simulink model "BD_PAR_SS"  (Simulink 10.3)
settings: Solver=ode1  StartTime=0.0  StopTime=max(cyc_mph(:,1))  FixedStep=1  MaxStep=1  RelTol=1e-3  AbsTol=1e-3
undefined symbols (not defined in the file): acc_elec_eff, acc_elec_pwr, acc_mech_eff, amb_tmp, cs_charge_deplete_bool, cs_electric_decel_spd, cs_electric_launch_spd_hi, cs_electric_launch_spd_lo, cs_hi_soc, cs_lo_soc, cs_off_trq_frac, cyc_avg_time, cyc_cargo_mass, cyc_elevation_init, cyc_filter_bool, cyc_grade, cyc_mph, ess_module_num, ess_on, ess_voc, ex_calc, ex_cat_co_frac, ex_cat_ext_cp, ex_cat_ext_emisv, ex_cat_ext_init_tmp, ex_cat_ext_mass, ex_cat_ext_sarea, ex_cat_hc_frac, ex_cat_i2p_th_cond, ex_cat_i2x_emisv, ex_cat_i2x_th_cond, ex_cat_int_cp, ex_cat_int_init_tmp, ex_cat_int_mass, ex_cat_int_sarea, ex_cat_lim, ex_cat_m2i_th_cond, ex_cat_m2i_tmp, ex_cat_m2p_emisv, ex_cat_mon_cp, ex_cat_mon_init_tmp, ex_cat_mon_mass, ex_cat_mon_sarea, ex_cat_monf_sarea, ex_cat_moni_sarea, ex_cat_nox_frac, ex_cat_p2x_th_cond, ex_cat_pcm_ecp, ex_cat_pcm_mass, ex_cat_pcm_tmp, ex_cat_pipe_cp, ex_cat_pipe_emisv, ex_cat_pipe_init_tmp, ex_cat_pipe_mass, ex_cat_pipe_sarea, ex_cat_pm_frac, ex_cat_tmp_range, ex_gas_cp, ex_manif_cp, ex_manif_emisv ... (+73)
libraries: lib_controls x6, lib_vehicle x3, lib_accessory x2, lib_interactive x1, lib_energy_storage x1, lib_fuel_converter x1
(part 4 of 6)

== system BD_PAR_SS/motor/ controller <mc> par/motor speed estimator ==
  mc_spd_out_a : Inport
  <= max spd : Saturate  UpperLimit=max(mc_map_spd)*mc_spd_scale  LowerLimit=-inf
  Block NOTES : Subsystem
      mask Display: disp('Block\nNOTES')
  Constant : Constant  Value=eps
  Constant1 : Constant  Value=0
  Constant2 : Constant  Value=2
  Gain : Gain  Gain=0.447  SaturateOnIntegerOverflow=on
  Logical Operator1 : Logic
  Memory : Memory  InitialCondition=cyc_mph(1,2)*0.447/wh_radius*fd_ratio*max(gb_ratio)*tc_mc_to_fc_ratio
  Memory1 : Memory  InitialCondition=1
  Memory2 : Memory
  Product : Product  Inputs=**/  SaturateOnIntegerOverflow=on
  Relational : RelationalOperator  Operator=>  RndMeth=Nearest  InputSameDT=on
  Relational Operator1 : RelationalOperator  Operator=~=  RndMeth=Nearest  InputSameDT=on
  Sum : Sum  SaturateOnIntegerOverflow=on
  Sum1 : Sum  Inputs=-+  SaturateOnIntegerOverflow=on
  Switch : Switch  Threshold=eps  SaturateOnIntegerOverflow=on  InputSameDT=on
  Switch1 : Switch  Threshold=eps  SaturateOnIntegerOverflow=on  InputSameDT=on
  To Workspace7 : ToWorkspace  VariableName=mc_spd_est  SampleTime=-1
  Out1 : Outport
  tag scope: mc_spd_limited=global
  wires:
  Switch/1 -> Memory/1
  Memory1/1 -> Switch1/2
  Relational/1 -> Memory1/1
  Sum1/1 -> Relational/1
  Constant2/1 -> Relational/2
  [mpha] -> Sum1/1, Gain/1
  [cyc_mph_r] -> Sum1/2
  Constant/1 -> Sum/2
  Memory/1 -> Switch1/1
  Constant1/1 -> Switch/3
  [veh_spd_a_rec] -> Switch/2, Sum/1
  Gain/1 -> Product/2
  Sum/1 -> Product/3
  Product/1 -> Switch/1
  mc_spd_out_a/1 -> Product/1, Switch1/3
  Memory2/1 -> Logical Operator1/2
  Logical Operator1/1 -> [mc_spd_limited]
  Relational Operator1/1 -> Logical Operator1/1, Memory2/1
  Switch1/1 -> <= max spd/1, Relational Operator1/1
  <= max spd/1 -> Out1/1, To Workspace7/1, Relational Operator1/2

== system BD_PAR_SS/motor/ controller <mc> par/rotor drive torque available (Nm) ==
  torque per unit input power (N-m/W) : Inport
  available input power (W) : Inport  Port=2
  Block NOTES : Subsystem
      mask Display: disp('Block\nNOTES')
  Constant2 : Constant  Value=inf
  Constant3 : Constant  Value=0
  Product : Product  SaturateOnIntegerOverflow=on
  Relational Operator : RelationalOperator  Operator=~=  RndMeth=Nearest  InputSameDT=on
  Switch : Switch  Threshold=eps  SaturateOnIntegerOverflow=on  InputSameDT=on
  rotor drive torque available : Outport  InitialOutput=0
  wires:
  torque per unit input power (N-m/W)/1 -> Relational Operator/1, Product/1
  Switch/1 -> rotor drive torque available/1
  Relational Operator/1 -> Switch/2
  Product/1 -> Switch/1
  available input power (W)/1 -> Product/2
  Constant2/1 -> Relational Operator/2
  Constant3/1 -> Switch/3

== system BD_PAR_SS/power bus <pb>/Block NOTES ==
  note: This power bus requires power from (or distributes power to)
      | the generator first, taking the balance from the energy
      | storage system.

== system BD_PAR_SS/torque coupler <tc>/Block NOTES ==
  note: speed, while the motor's speed may be different.  The ratio of motor speed to main
      | output speed is stored in the variable tc_mc_to_fc_spd_ratio.
  note: This block models a chain- or belt-driven torque coupler, with three gears:  one each
      | for the motor, main input (the engine or gearbox), and main output (to the gearbox
      | or final drive).  It includes losses in the chain or belt, but leaves inertia effects to be
      | considered in the appropriate component.
      |
      | The entire torque required out of the torque coupler (plus losses) is required from the
      | engine.  The engine provides only as much torque as its engine controller (see the
      | <vc> block) allows.  Any remaining unmet torque request is submitted to the motor,
      | which meets the request to the best of its ability.
      |
      | The torque converter output speed is limited by the maximum speeds of both the
      | motor and the engine.
      |
      | The loss torque is zero when the gears are not turning, and is applied at the output
      |  gear.
      |
      | The gears connecting the main input and main output to the torque converter's belt
      | or chain are assumed to be of the same size, so that main input speed = main output

== system BD_PAR_SS/torque coupler <tc>/help ==

== system BD_PAR_SS/torque coupler <tc>/loss (Nm) ==
  note: The loss torque is zero when the gears are not turning,
      | and is applied at the torque coupler's output gear.
  tc output speed (rad/s) : Inport
  Constant : Constant  Value=0
  Switch : Switch  Threshold=eps  SaturateOnIntegerOverflow=on  InputSameDT=on
  torque coupler loss torque (Nm) : Constant  Value=tc_loss
  drag torque (Nm) : Outport  InitialOutput=0
  wires:
  torque coupler loss torque (Nm)/1 -> Switch/1
  Switch/1 -> drag torque (Nm)/1
  tc output speed (rad/s)/1 -> Switch/2
  Constant/1 -> Switch/3

== system BD_PAR_SS/vehicle <veh>/Block NOTES ==
  note: A slight simplification, the assumption that (speed_at_end_of_time_step)^2 is roughly equal to
      | (speed_at_end_of_time_step)*(speed_at_beginning_of_time_step), is used to avoid solving
      | a quadratic equation in the solution of v=v(Ftract).
  note: This block uses the required vehicle speed with vehicle parameters and the previous speed
      | and classic, straightforward equations to determine the tractive force required at the tire/road interface.
  note: If no drivetrain component ran up against its performance limit during the time step, the achieved speed
      | is taken to be the requested speed.
  note: Given the tractive force available, this block uses the same equations to determine the achievable speed.

== system BD_PAR_SS/vehicle <veh>/force req'd to accelerate (N) ==
  v(m/s) : Inport
  v prev : Inport  Port=2
  Clock : Clock
  Memory : Memory  InitialCondition=-0.1
  Product1 : Product  Inputs=**/  SaturateOnIntegerOverflow=on
  Sum : Sum  Inputs=+-  SaturateOnIntegerOverflow=on
  Sum1 : Sum  Inputs=+-  SaturateOnIntegerOverflow=on
  current veh mass : Subsystem
  (N) : Outport  InitialOutput=0
  wires:
  current veh mass/1(Out1) -> Product1/1
  Clock/1 -> Sum1/1, Memory/1
  Memory/1 -> Sum1/2
  Product1/1 -> (N)/1
  v prev/1 -> Sum/2
  v(m/s)/1 -> Sum/1
  Sum1/1 -> Product1/3
  Sum/1 -> Product1/2

== system BD_PAR_SS/vehicle <veh>/force req'd to ascend (N) ==
  average vehicle speed over time step (m/s) : Inport
  Constant : Constant  Value=veh_gravity
  Constant1 : Constant  Value=0
  Product : Product  Inputs=3  SaturateOnIntegerOverflow=on
  Switch : Switch  SaturateOnIntegerOverflow=on  InputSameDT=on
  Trigonometric Function : Trigonometry  Operator=atan
  Trigonometric Function1 : Trigonometry
  current veh mass : Subsystem
  (N) : Outport  InitialOutput=0
  wires:
  current veh mass/1(Out1) -> Product/3
  average vehicle speed over time step (m/s)/1 -> Switch/2
  Constant1/1 -> Switch/3
  Switch/1 -> (N)/1
  Product/1 -> Switch/1
  Constant/1 -> Product/1
  [grade] -> Trigonometric Function/1
  Trigonometric Function1/1 -> Product/2
  Trigonometric Function/1 -> Trigonometric Function1/1

== system BD_PAR_SS/vehicle <veh>/force req'd to overcome aerodynamic drag (N) ==
  average vehicle speed over time step (m/s) : Inport
  Constant : Constant  Value=veh_air_density*veh_CD*veh_FA*0.5
  Product : Product  Inputs=3  SaturateOnIntegerOverflow=on
  D aero(N) : Outport  InitialOutput=0
  wires:
  Product/1 -> D aero(N)/1
  Constant/1 -> Product/3
  average vehicle speed over time step (m/s)/1 -> Product/2, Product/1

== system BD_PAR_SS/vehicle <veh>/help ==

== system BD_PAR_SS/vehicle <veh>/record achieved force outputs ==
  spd_prev : Inport
  spd : Inport  Port=2
  Gain1 : Gain  Gain=0.5  SaturateOnIntegerOverflow=on
  Product{,1..3} (4 alike) : Product  SaturateOnIntegerOverflow=on
  Sum2 : Sum  SaturateOnIntegerOverflow=on
  To Workspace1 : ToWorkspace  VariableName=veh_pwr_rr_a  SampleTime=-1
  To Workspace4 : ToWorkspace  VariableName=veh_pwr_accel_a  SampleTime=-1
  To Workspace6 : ToWorkspace  VariableName=veh_pwr_drag_a  SampleTime=-1
  To Workspace7 : ToWorkspace  VariableName=veh_pwr_ascent_a  SampleTime=-1
  force req'd to accelerate (N)1 : Subsystem
  force req'd to ascend (N)1 : Subsystem
  force req'd to overcome aerodynamic drag (N)1 : Subsystem
  rolling resistance force : Subsystem  BlockChoice=force req'd to overcome rolling resistance (N)
      settings: AttributesFormatString=%<BlockChoice>  TemplateBlock=lib_vehicle/Submodels/rolling resistance force  MemberBlocks=force req'd to overcome rolling resistance (N),force req'd to overcome rolling resistance (N) j2452
  tag scope: veh_pwr_accel_a=global, veh_pwr_ascent_a=global, veh_pwr_drag_a=global, veh_pwr_rr_a=global
  wires:
  Gain1/1 -> [vel_ave], rolling resistance force/1(average vehicle speed over time step (m/s)), force req'd to ascend (N)1/1(average vehicle speed over time step (m/s)), force req'd to overcome aerodynamic drag (N)1/1(average vehicle speed over time step (m/s))
  Product3/1 -> To Workspace1/1, [veh_pwr_rr_a]
  [vel_ave] -> Product3/2
  Product2/1 -> [veh_pwr_ascent_a], To Workspace7/1
  [vel_ave] -> Product2/2
  [vel_ave] -> Product1/2
  [vel_ave] -> Product/2
  Product1/1 -> [veh_pwr_drag_a], To Workspace6/1
  Product/1 -> [veh_pwr_accel_a], To Workspace4/1
  force req'd to accelerate (N)1/1((N)) -> Product/1
  rolling resistance force/1(Fr (N)) -> Product3/1
  force req'd to ascend (N)1/1((N)) -> Product2/1
  force req'd to overcome aerodynamic drag (N)1/1(D aero(N)) -> Product1/1
  spd_prev/1 -> Sum2/2, force req'd to accelerate (N)1/2(v prev)
  spd/1 -> Sum2/1, force req'd to accelerate (N)1/1(v(m/s))
  Sum2/1 -> Gain1/1

== system BD_PAR_SS/vehicle <veh>/rolling resistance force ==
  average vehicle speed over time step (m/s) : Inport
  force req'd to overcome rolling resistance (N) : lib_vehicle/Submodels/force req'd to overcome rolling resistance (N)  SystemSampleTime=-1  VariantActivationTime=update diagram  Latency=0  AutoFrameSizeCalculation=off
  Fr (N) : Outport
  wires:
  average vehicle speed over time step (m/s)/1 -> force req'd to overcome rolling resistance (N)/1
  force req'd to overcome rolling resistance (N)/1 -> Fr (N)/1

== system BD_PAR_SS/vehicle <veh>/vehicle speed ==
  vehicle speed at beginning of time step (m/s) : Inport
  "available tractive force and linear speed (N), (m/s)" : Inport  Port=2
  vehicle speed (m/s) : lib_vehicle/Submodels/vehicle speed (m//s)  SystemSampleTime=-1  VariantActivationTime=update diagram  Latency=0  AutoFrameSizeCalculation=off
  vehicle speed achievable at end of time step (m/s) : Outport
  wires:
  vehicle speed at beginning of time step (m/s)/1 -> vehicle speed (m/s)/1
  "available tractive force and linear speed (N), (m/s)"/1 -> vehicle speed (m/s)/2
  vehicle speed (m/s)/1 -> vehicle speed achievable at end of time step (m/s)/1

== system BD_PAR_SS/wheel and axle  front/rear <wh>/Block NOTES ==
  note: This block determines the required axle torque and speed given the tractive force and
      | speed required to meet the trace in the top blocks, and determines the available tractive
      | force and possible vehicle speed given the drivetrain-input torque and rotational speed
      | in the bottom blocks.  The "wheel control" blocks apply the braking strategy and ensure
      | that accelerations beyond the capability of the tires are not requested.

== system BD_PAR_SS/wheel and axle  front/rear <wh>/effect of  inertia (Nm) ==
  note: This block computes the torque required to overcome the inertia of the
      | wheels and axle.
  axle input speed (rad/s) : Inport
  Constant : Constant  Value=wh_inertia
  Product : Product  SaturateOnIntegerOverflow=on
  d/dt : Derivative
  inertia torque (Nm) : Outport  InitialOutput=0
  wires:
  Product/1 -> inertia torque (Nm)/1
  Constant/1 -> Product/2
  axle input speed (rad/s)/1 -> d/dt/1
  d/dt/1 -> Product/1

== system BD_PAR_SS/wheel and axle  front/rear <wh>/front brake ==
  F_brake : Inport
  Constant : Constant  Value=wh_max_front_brake_force
  Terminator : Terminator
  F_brake_max : Outport  InitialOutput=0
  wires:
  Constant/1 -> F_brake_max/1
  F_brake/1 -> Terminator/1

== system BD_PAR_SS/wheel and axle  front/rear <wh>/front force ==
  In1 : Inport
  In2 : Inport  Port=2
  Product1 : Product  SaturateOnIntegerOverflow=on
  Sum2 : Sum  Inputs=-+  SaturateOnIntegerOverflow=on
  To Workspace12 : ToWorkspace  VariableName=wh_front_brake_r  SampleTime=-1
  brake request  controller interface : Subsystem
  tractive torque req/d of drivetrain (Nm) : Gain  Gain=wh_radius  SaturateOnIntegerOverflow=on
  Out1 : Outport
  wires:
  tractive torque req/d of drivetrain (Nm)/1 -> Out1/1
  In2/1 -> Product1/2
  In1/1 -> Product1/1
  Product1/1 -> Sum2/2
  Sum2/1 -> tractive torque req/d of drivetrain (Nm)/1
  brake request  controller interface/1(F_front_brake_req) -> To Workspace12/1, Sum2/1

== system BD_PAR_SS/wheel and axle  front/rear <wh>/front/rear brake controller interface (achievable) ==
  F_drivetrain_ach : Inport
  w_wheel_ach : Inport  Port=2
  F_rear_drivetrain_ach : Inport  Port=3
  F_max_front_brake : Inport  Port=4
  F_max_rear_brake : Inport  Port=5
  F_front_brake : Outport  InitialOutput=0
  F_rear_brake : Outport  Port=2  InitialOutput=0
  tag scope: F_drivetrain_ach=global, F_max_front_brake=global, F_max_rear_brake=global, F_rear_drivetrain_ach=global, w_wheel_ach=global
  wires:
  F_rear_drivetrain_ach/1 -> [F_rear_drivetrain_ach]
  F_max_rear_brake/1 -> [F_max_rear_brake]
  F_max_front_brake/1 -> [F_max_front_brake]
  F_drivetrain_ach/1 -> [F_drivetrain_ach]
  w_wheel_ach/1 -> [w_wheel_ach]
  [F_front_brake] -> F_front_brake/1
  [F_rear_brake] -> F_rear_brake/1

== system BD_PAR_SS/wheel and axle  front/rear <wh>/help ==

== system BD_PAR_SS/wheel and axle  front/rear <wh>/limits and losses diagnostics ==
  speed : Inport
  front brake : Inport  Port=2
  front brake max : Inport  Port=3
  rear brake max : Inport  Port=4
  rear brake : Inport  Port=5
  Gain : Gain  Gain=-1  SaturateOnIntegerOverflow=on
  Logical Operator : Logic  Operator=OR
  Product : Product  SaturateOnIntegerOverflow=on
  Relational Operator1 : RelationalOperator  Operator===  RndMeth=Nearest  InputSameDT=on
  Relational Operator2 : RelationalOperator  Operator===  RndMeth=Nearest  InputSameDT=on
  Sum3 : Sum  SaturateOnIntegerOverflow=on
  To Workspace6 : ToWorkspace  VariableName=wh_brake_loss_pwr  SampleTime=-1
  tag scope: brake_limited=global
  wires:
  rear brake/1 -> Relational Operator2/2, Sum3/2
  rear brake max/1 -> Relational Operator2/1
  front brake max/1 -> Relational Operator1/2
  front brake/1 -> Relational Operator1/1, Sum3/1
  speed/1 -> Product/1
  Relational Operator2/1 -> Logical Operator/2
  Relational Operator1/1 -> Logical Operator/1
  Logical Operator/1 -> [brake_limited]
  Product/1 -> To Workspace6/1
  Sum3/1 -> Gain/1
  Gain/1 -> Product/2

== system BD_PAR_SS/wheel and axle  front/rear <wh>/loss (Nm) ==
  note: The loss torque is zero when the axle is not turning.
  axle speed (rad/s) : Inport
  Constant : Constant  Value=0
  Switch : Switch  Threshold=eps  SaturateOnIntegerOverflow=on  InputSameDT=on
  veh mass calc : Subsystem
  wheel & axle bearing drag (Nm) : Lookup  InputValues=wh_axle_loss_mass  Table=wh_axle_loss_trq  SaturateOnIntegerOverflow=on
  drag torque (Nm) : Outport  InitialOutput=0
  wires:
  wheel & axle bearing drag (Nm)/1 -> Switch/1
  Constant/1 -> Switch/3
  axle speed (rad/s)/1 -> Switch/2
  Switch/1 -> drag torque (Nm)/1
  veh mass calc/1(Out1) -> wheel & axle bearing drag (Nm)/1

== system BD_PAR_SS/wheel and axle  front/rear <wh>/rear brake ==
  F_brake : Inport
  Constant : Constant  Value=wh_max_rear_brake_force
  Terminator : Terminator
  F_brake_max : Outport  InitialOutput=0
  wires:
  F_brake/1 -> Terminator/1
  Constant/1 -> F_brake_max/1

== system BD_PAR_SS/wheel and axle  front/rear <wh>/rear force ==
  In1 : Inport
  In2 : Inport  Port=2
  Product2 : Product  SaturateOnIntegerOverflow=on
  Sum1 : Sum  Inputs=-+  SaturateOnIntegerOverflow=on
  Sum4 : Sum  Inputs=-+  SaturateOnIntegerOverflow=on
  To Workspace12 : ToWorkspace  VariableName=wh_rear_brake_r  SampleTime=-1
  brake request controller interface1 : Subsystem
  tractive torque req/d of drivetrain (Nm)1 : Gain  Gain=wh_radius  SaturateOnIntegerOverflow=on
  Out1 : Outport
  wires:
  Sum1/1 -> Sum4/2
  Product2/1 -> Sum1/1
  In2/1 -> Product2/2
  In1/1 -> Sum1/2, Product2/1
  tractive torque req/d of drivetrain (Nm)1/1 -> Out1/1
  Sum4/1 -> tractive torque req/d of drivetrain (Nm)1/1
  brake request controller interface1/1(F_rear_brake_req) -> To Workspace12/1, Sum4/1

== system BD_PAR_SS/wheel and axle  front/rear <wh>/tire slip model (m/s) ==
  note: See note regarding sum in backward path
  weight borne  by front axle (N) : Inport
  total tractive  force available (N) : Inport  Port=2
  axle speed available (rad/s) : Inport  Port=3
  axle speed req'd (rad/s) : Inport  Port=4
  vehicle speed required (m/s) : Inport  Port=5
  weight borne by  rear axle (N) : Inport  Port=6
  front fraction : Inport  Port=7
  Abs1 : Abs  SaturateOnIntegerOverflow=on
  Block NOTES : Subsystem
      mask Display: disp('Block\nNOTES')
  Constant : Constant  Value=1e-3
  Constant5 : Constant
  Constant6 : Constant  Value=wh_radius
  Fcn : Fcn  Expr=1/u
  Relational Operator1 : RelationalOperator  Operator=>  RndMeth=Nearest  InputSameDT=on
  Sum1 : Sum  Inputs=+-  SaturateOnIntegerOverflow=on
  Sum2 : Sum  SaturateOnIntegerOverflow=on
  Sum3 : Sum  SaturateOnIntegerOverflow=on
  Sum4 : Sum  Inputs=-+  SaturateOnIntegerOverflow=on
  Switch1 : Switch  Threshold=eps  SaturateOnIntegerOverflow=on  InputSameDT=on
  front axle : Subsystem
  front frac : Product  SaturateOnIntegerOverflow=on
  rear axle : Subsystem
  vehicle speed (m/s) : Product  Inputs=3  SaturateOnIntegerOverflow=on
  possible vehicle speed (m/s) : Outport  InitialOutput=0
  tag scope: veh_spd_a_rec=global
  wires:
  Sum2/1 -> Sum3/1
  rear axle/1(Out1) -> Sum2/2
  front axle/1(Out1) -> Sum2/1
  Sum1/1 -> rear axle/2(In2)
  front frac/1 -> Sum1/2, front axle/2(In2)
  front fraction/1 -> front frac/2
  total tractive  force available (N)/1 -> Sum1/1, front frac/1
  weight borne by  rear axle (N)/1 -> rear axle/1(In1)
  vehicle speed (m/s)/1 -> [veh_spd_a_rec], Switch1/1
  Switch1/1 -> possible vehicle speed (m/s)/1
  weight borne  by front axle (N)/1 -> front axle/1(In1)
  Abs1/1 -> Relational Operator1/1
  Constant/1 -> Relational Operator1/2
  axle speed req'd (rad/s)/1 -> Sum4/2
  Sum4/1 -> Abs1/1
  vehicle speed required (m/s)/1 -> Switch1/3
  Relational Operator1/1 -> Switch1/2
  Constant6/1 -> vehicle speed (m/s)/3
  axle speed available (rad/s)/1 -> vehicle speed (m/s)/2, Sum4/1
  Constant5/1 -> Sum3/2
  Fcn/1 -> vehicle speed (m/s)/1
  Sum3/1 -> Fcn/1

== system BD_PAR_SS/wheel and axle  front/rear <wh>/tire slip model (rad/s) ==
  note: Question: for front and rear, is it the sum of or min/max? tm:020703
  note: This block implements the effects of finite tire slip
      | (with respect to the road) on the vehicle speed/wheel speed relationship.
  note: Slip is defined as s=(omega*r - v) / v.  The one-to-one mapping of slip to normalized
      | tractive force, F_tract/W_front_axle, up to the maximum, is stored in the variables
      | "wh_slip" and "wh_slip_force_coeff."
  total tractive  force requested (N) : Inport
  requested time-step average vehicle speed (m/s) : Inport  Port=2
  weight borne by front axle (N) : Inport  Port=3
  weight borne by  rear axle (N)1 : Inport  Port=4
  front traction ratio : Inport  Port=5
  Constant5 : Constant
  Constant6 : Constant  Value=1/wh_radius
  Sum1 : Sum  Inputs=+-  SaturateOnIntegerOverflow=on
  Sum2 : Sum  SaturateOnIntegerOverflow=on
  Sum3 : Sum  SaturateOnIntegerOverflow=on
  To Workspace6 : ToWorkspace  VariableName=wh_slip_r  SampleTime=-1
  front frac : Product  SaturateOnIntegerOverflow=on
  front slip : Subsystem
  rear slip : Subsystem
  wheel speed (rad/s) : Product  Inputs=3  SaturateOnIntegerOverflow=on
  slip-augmented rotational speed (rad/s) : Outport  InitialOutput=0
  wires:
  Sum2/1 -> To Workspace6/1, Sum3/1
  rear slip/1(Out1) -> Sum2/2
  front slip/1(Out1) -> Sum2/1
  weight borne by  rear axle (N)1/1 -> rear slip/1(In1)
  Sum1/1 -> rear slip/2(In2)
  front traction ratio/1 -> front frac/2
  total tractive  force requested (N)/1 -> Sum1/1, front frac/1
  front frac/1 -> front slip/2(In2), Sum1/2
  wheel speed (rad/s)/1 -> slip-augmented rotational speed (rad/s)/1
  Constant5/1 -> Sum3/2
  Sum3/1 -> wheel speed (rad/s)/2
  Constant6/1 -> wheel speed (rad/s)/3
  requested time-step average vehicle speed (m/s)/1 -> wheel speed (rad/s)/1
  weight borne by front axle (N)/1 -> front slip/1(In1)

== system BD_PAR_SS/wheel and axle  front/rear <wh>/traction controller interface ==
  F_req : Inport
  v_ave_req : Inport  Port=2
  F_req_limited : Outport  InitialOutput=0
  v_req_limited : Outport  Port=2  InitialOutput=0
  wt_front_axle : Outport  Port=3  InitialOutput=0
  wt_rear_axle : Outport  Port=4  InitialOutput=0
  front_traction_ratio : Outport  Port=5  InitialOutput=0
  tag scope: F_req=global, v_ave_req=global
  wires:
  [front_traction_ratio] -> front_traction_ratio/1
  [wt_rear_axle] -> wt_rear_axle/1
  v_ave_req/1 -> [v_ave_req]
  F_req/1 -> [F_req]
  [wt_front_axle] -> wt_front_axle/1
  [v_req_limited] -> v_req_limited/1
  [F_req_limited] -> F_req_limited/1

== system BD_PAR_SS/<vc> par/engine on (parallel hybrid)/Block NOTES1 ==
  note: This engine state computer keeps the engine on if:
      | [
      | 1) key is on, AND
      | 2) (trq is too high AND speed is too high for idle) OR engine is allowed to idle, AND
      | 3) vehicle speed >= cs_electric_launch_spd [ in m/s ], AND
      | 4) req'd trq > (cs_off_trq_frac * max_trq_at_spd) OR SOC<cs_lo_soc
      | ]
      | OR
      | [ engine was previously on AND the transmission is shifting ]
      |
      | The last condition is added to prevent the engine from unrealistically
      | shutting down for a second or two during a shift.

== system BD_PAR_SS/<vc> par/engine on (parallel hybrid)/Subsystem ==
  in_1 : Inport
  Clock : Clock
  Constant1 : Constant  Value=n
  Constant2 : Constant
  Integrator : Integrator
  Memory : Memory  InitialCondition=-0.1
  Memory1 : Memory
  Product : Product  Inputs=*/  InputSameDT=on  RndMeth=Zero  SaturateOnIntegerOverflow=on  OutDataTypeStr=Inherit: Same as first input
  Product1 : Product  InputSameDT=on  RndMeth=Zero  SaturateOnIntegerOverflow=on  OutDataTypeStr=Inherit: Same as first input
  Relational Operator : RelationalOperator  Operator=<=  RndMeth=Nearest  InputSameDT=on
  Sum : Sum  Inputs=+-  InputSameDT=on  SaturateOnIntegerOverflow=on  OutDataTypeStr=Inherit: Same as first input
  Sum1 : Sum  Inputs=|+-  InputSameDT=on  SaturateOnIntegerOverflow=on  OutDataTypeStr=Inherit: Same as first input
  Switch{,1..3} (4 alike) : Switch  Threshold=eps  SaturateOnIntegerOverflow=on  InputSameDT=on
  Variable Transport Delay : VariableTransportDelay  MaximumDelay=n  ZeroDelay=on
  out_1 : Outport  InitialOutput=0
  wires:
  Product/1 -> out_1/1
  Sum/1 -> Product/1
  Variable Transport Delay/1 -> Sum/2
  Integrator/1 -> Variable Transport Delay/1, Sum/1
  Relational Operator/1 -> Switch/2
  Constant1/1 -> Product1/2
  Clock/1 -> Sum1/1, Memory/1, Relational Operator/1, Switch/1
  Memory/1 -> Sum1/2
  Sum1/1 -> Product1/1
  Product1/1 -> Relational Operator/2, Switch/3
  Switch/1 -> Variable Transport Delay/2, Switch1/2, Switch1/1
  Constant2/1 -> Switch1/3
  Switch1/1 -> Product/2
  Switch2/1 -> Integrator/1
  Switch3/1 -> Memory1/1
  in_1/1 -> Switch2/3, Switch3/3
  Memory1/1 -> Switch2/1, Switch3/1
  [shifting] -> Switch2/2, Switch3/2

== system BD_PAR_SS/<vc> par/engine on (parallel hybrid)/key_on ==
  Clock : Clock
  Fcn1 : Fcn  Expr=rem(u[1],period)
  Look-Up Table : Lookup  InputValues=t  Table=y  SaturateOnIntegerOverflow=on
  out_1 : Outport  InitialOutput=0
  wires:
  Fcn1/1 -> Look-Up Table/1
  Clock/1 -> Fcn1/1
  Look-Up Table/1 -> out_1/1

== system BD_PAR_SS/<vc> par/engine on (parallel hybrid)/repeated cycle:  speed required at end of NEXT step ==
  Clock : Clock
  Fcn1 : Fcn  Expr=rem(u[1],period)
  Look-Up Table : Lookup  InputValues=t  Table=y  SaturateOnIntegerOverflow=on
  Memory : Memory  InitialCondition=-0.1
  Sum : Sum  Inputs=+-  InputSameDT=on  SaturateOnIntegerOverflow=on  OutDataTypeStr=Inherit: Same as first input
  Sum1 : Sum  InputSameDT=on  SaturateOnIntegerOverflow=on  OutDataTypeStr=Inherit: Same as first input
  out_1 : Outport  InitialOutput=0
  wires:
  Sum1/1 -> Look-Up Table/1
  Look-Up Table/1 -> out_1/1
  Fcn1/1 -> Sum1/1
  Sum/1 -> Sum1/2
  Memory/1 -> Sum/2
  Clock/1 -> Fcn1/1, Memory/1, Sum/1

== system BD_PAR_SS/<vc> par/motor controller logic/Block NOTES ==
  note: This block models a motor/controller's logic, modulating the power input requirement as follows:
      | - enforcing the maximum current limit of the motor/controller
      | - shutting the motor off if the average speed over the time step ==0
      | - shutting the motor off if the transmission is shifting.

== system BD_PAR_SS/<vc> par/motor controller logic/Sign ==
  in_1 : Inport
  Constant : Constant  Value=0
  Relational Operator : RelationalOperator  Operator=>  RndMeth=Nearest  InputSameDT=on
  Relational Operator1 : RelationalOperator  Operator=<  RndMeth=Nearest  InputSameDT=on
  Sum : Sum  Inputs=+-  InputSameDT=on  SaturateOnIntegerOverflow=on  OutDataTypeStr=Inherit: Same as first input
  out_1 : Outport  InitialOutput=0
  wires:
  Sum/1 -> out_1/1
  Relational Operator/1 -> Sum/1
  Relational Operator1/1 -> Sum/2
  Constant/1 -> Relational Operator/2, Relational Operator1/2
  in_1/1 -> Relational Operator1/1, Relational Operator/1

== system BD_PAR_SS/<vc> par/parallel clutch control/Block NOTES ==
  note: This clutch control block determines the clutch state given the req'd clutch output torque
      | and speed (labelled as gearbox input torque and speed), and the gear number history.
      |                           conditions                                                                       clutch state
      | gear is being shifted OR (trq <~ 0 AND (engine is                                     1 == disengaged
      | clutched to avoid compression braking OR spd < idle))
      |
      | (trq >~ 0) AND (spd < launch speed) AND clutch                                       2 == slipping
      | was not engaged during previous time step
      |
      | neither of above sets of conditions are met                                          3 == engaged
      |
      | But the clutch is always disengaged when the engine is off or was off within the past 0.5 s.

== system BD_PAR_SS/<vc> par/parallel clutch control/gearbox speed estimator ==
  gb_spd_in_r if no gear change : Inport
  Block NOTES : Subsystem
      mask Display: disp('Block\nNOTES')
  Constant : Constant  Value=eps
  Constant1 : Constant  Value=0
  Constant2 : Constant
  Constant3 : Constant  Value=0.11
  Gain : Gain  Gain=0.447  SaturateOnIntegerOverflow=on  OutDataTypeStr=Inherit: Same as input  ParamDataTypeStr=Inherit: Same as input
  Logical : Logic
  Memory : Memory  InitialCondition=cyc_mph(1,2)*0.447/wh_radius*fd_ratio*gb_ratio(gb_num_init)
  Memory1 : Memory  InitialCondition=1
  Product : Product  Inputs=**/  InputSameDT=on  RndMeth=Zero  SaturateOnIntegerOverflow=on  OutDataTypeStr=Inherit: Same as first input
  Relational : RelationalOperator  Operator=>  RndMeth=Nearest  InputSameDT=on
  Relational1 : RelationalOperator  Operator=<=  RndMeth=Nearest  InputSameDT=on
  Sum : Sum  InputSameDT=on  SaturateOnIntegerOverflow=on  OutDataTypeStr=Inherit: Same as first input
  Sum1 : Sum  Inputs=-+  InputSameDT=on  SaturateOnIntegerOverflow=on  OutDataTypeStr=Inherit: Same as first input
  Switch : Switch  Threshold=eps  SaturateOnIntegerOverflow=on  InputSameDT=on
  Switch1 : Switch  Threshold=eps  SaturateOnIntegerOverflow=on  InputSameDT=on
  dt : Subsystem
  Out1 : Outport
  wires:
  Product/1 -> Switch/1
  Sum/1 -> Product/3
  Gain/1 -> Product/2
  [veh_spd_a_rec] -> Sum/1, Switch/2
  Constant1/1 -> Switch/3
  Memory/1 -> Switch1/1
  Constant/1 -> Sum/2
  [cyc_mph_r] -> Sum1/2
  [mpha] -> Gain/1, Sum1/1
  Constant2/1 -> Relational/2
  Sum1/1 -> Relational/1
  Relational/1 -> Memory1/1
  Switch/1 -> Memory/1
  Switch1/1 -> Out1/1
  gb_spd_in_r if no gear change/1 -> Switch1/3
  [gb_spd_in_a] -> Product/1
  Constant3/1 -> Relational1/2
  Relational1/1 -> Logical/2
  Memory1/1 -> Logical/1
  Logical/1 -> Switch1/2
  dt/1(Out1) -> Relational1/1

== system BD_PAR_SS/<vc> par/pre-TX parallel gearbox control/Block NOTES ==
  note: This gearbox control block computes the current gear number given the gearbox's
      | req'd output torque and speed and an estimate its efficiency.  Upshifts occur, given a
      | certain engine speed,  when the estimated engine load falls below the upshift curve
      | in engine speed/load space, and downshifts likewise occur when estimated engine
      | load rises above the downshift curve.  Separate upshift and downshift curves are
      | defined for each gear.  An upshift may not be immediately followed by a downshift.
      | If the tires are about to slip, don't upshift unless the engine would be at max. speed.
      | Enforce this rule by setting the load to 1 when the tires are about to slip.

== system BD_PAR_SS/<vc> par/pre-TX parallel gearbox control/allow downshift? ==
  prev gearnum : Inport
  Logical Operator : Logic  Operator=NOR
  Memory : Memory  InitialCondition=1
  Memory1 : Memory  InitialCondition=1
  Relational Operator1 : RelationalOperator  Operator=>  RndMeth=Nearest  InputSameDT=on
  Relational Operator2 : RelationalOperator  Operator=>  RndMeth=Nearest  InputSameDT=on
  allow shift : Outport  InitialOutput=0
  wires:
  Logical Operator/1 -> allow shift/1
  prev gearnum/1 -> Relational Operator1/1, Memory/1, Relational Operator2/1
  Relational Operator1/1 -> Logical Operator/1
  Memory/1 -> Relational Operator1/2, Memory1/1
  Memory1/1 -> Relational Operator2/2
  Relational Operator2/1 -> Logical Operator/2

== system BD_PAR_SS/<vc> par/pre-TX parallel gearbox control/allow upshift? ==
  prev gearnum : Inport
  gb_trq_out_r : Inport  Port=2
  gb_spd_out_r : Inport  Port=3
  prev Pout/Pin : Inport  Port=4
  Block NOTES1 : Subsystem
      mask Display: disp('Block\nNOTES')
  Constant : Constant
  Constant1 : Constant  Value=max(mc_map_spd)*mc_spd_scale/tc_mc_to_fc_ratio*.95
  Logical Operator1 : Logic  Operator=OR  Inputs=3
  Memory : Memory  InitialCondition=1
  Product : Product  InputSameDT=on  RndMeth=Zero  SaturateOnIntegerOverflow=on  OutDataTypeStr=Inherit: Same as first input
  Relational Operator : RelationalOperator  Operator=>  RndMeth=Nearest  InputSameDT=on
  Relational Operator1 : RelationalOperator  Operator=>  RndMeth=Nearest  InputSameDT=on
  Saturation : Saturate  UpperLimit=gb_gears_num  LowerLimit=1
  Sum : Sum  InputSameDT=on  SaturateOnIntegerOverflow=on  OutDataTypeStr=Inherit: Same as first input
  est. req'd input pwr (W) : Product  Inputs=**/  InputSameDT=on  RndMeth=Zero  SaturateOnIntegerOverflow=on  OutDataTypeStr=Inherit: Same as first input
  gear ratio : Lookup  InputValues=[1:length(gb_ratio)]  Table=gb_ratio  SaturateOnIntegerOverflow=on
  gear ratio1 : Lookup  InputValues=[1:length(gb_ratio)]  Table=gb_ratio  SaturateOnIntegerOverflow=on
  motor torque capability : Lookup  InputValues=mc_map_spd*mc_spd_scale  Table=mc_max_trq*mc_trq_scale*mc_overtrq_factor+eps  SaturateOnIntegerOverflow=on
  motor (input to gb) pwr capability : Product  InputSameDT=on  RndMeth=Zero  SaturateOnIntegerOverflow=on  OutDataTypeStr=Inherit: Same as first input
  req'd input spd if no gear change : Product  InputSameDT=on  RndMeth=Zero  SaturateOnIntegerOverflow=on  OutDataTypeStr=Inherit: Same as first input
  allow shift : Outport  InitialOutput=0
  wires:
  req'd input spd if no gear change/1 -> Relational Operator1/1
  Constant1/1 -> Relational Operator1/2
  Relational Operator1/1 -> Logical Operator1/3
  gb_spd_out_r/1 -> req'd input spd if no gear change/2, Product/2, est. req'd input pwr (W)/1
  prev gearnum/1 -> gear ratio1/1, Sum/1
  gear ratio1/1 -> req'd input spd if no gear change/1
  Constant/1 -> Sum/2
  Sum/1 -> Saturation/1
  Saturation/1 -> gear ratio/1
  gear ratio/1 -> Product/1
  motor torque capability/1 -> motor (input to gb) pwr capability/2
  Product/1 -> motor torque capability/1, motor (input to gb) pwr capability/1
  motor (input to gb) pwr capability/1 -> Relational Operator/1
  est. req'd input pwr (W)/1 -> Relational Operator/2
  gb_trq_out_r/1 -> est. req'd input pwr (W)/2
  prev Pout/Pin/1 -> est. req'd input pwr (W)/3
  Logical Operator1/1 -> allow shift/1
  Relational Operator/1 -> Logical Operator1/1
  [engine_on] -> Memory/1
  Memory/1 -> Logical Operator1/2

== system BD_PAR_SS/<vc> par/pre-TX parallel gearbox control/downshift  command ==
  prev gear number : Inport
  engine load : Inport  Port=2
  engine speed : Inport  Port=3
  Mux : Mux  Inputs=2
  Relational Operator : RelationalOperator  Operator=>  RndMeth=Nearest  InputSameDT=on
  load fraction : Subsystem  mask(Gear Selector){spd=gb_dnshift_spd, load=gb_dnshift_load}
      mask prompts: spd "Speeds:"; load "Load Fractions:"
      mask help:
      | This block will perform a linear interplation (extrapolation outside of bounds) to determine the shift point load fraction associated with the current gear number and speed.
      |
      | The Speeds parameter should be defined as an array of vectors containing speeds for each gear number.  The Load Fractions parameter should be defined as a array of vectors containing load fractions indexed by the speeds in the Speeds parameter for each gear number.
      mask Help:
      | Reference the base workspace variables - gb_**shift_spd and gb_**shift_load  where ** is either up for upshift conditions or dn for downshift conditions.
      | 
      | Or define the arrays as follows:
      | 
      | {[spd1 spd2 spd3 spd4]; [spd1 spd2 spd3 spd4]; ...}
      | 
      | {[load1 load2 load3 load4]; [load1 load2 load3 load4]; ...}
      | 
      | where each array contains one row for each gear in the gearbox.  Speeds should be defined in rad/s and loads as a decimal fraction.
  command : Outport  InitialOutput=0
  wires:
  Relational Operator/1 -> command/1
  engine speed/1 -> Mux/2
  prev gear number/1 -> Mux/1
  engine load/1 -> Relational Operator/1
  Mux/1 -> load fraction/1(In1)
  load fraction/1(Out1) -> Relational Operator/2

== system BD_PAR_SS/<vc> par/pre-TX parallel gearbox control/gearbox speed estimator ==
  gb_spd_in_r if no gear change : Inport
  Block NOTES : Subsystem
      mask Display: disp('Block\nNOTES')
  Constant : Constant  Value=eps
  Constant1 : Constant  Value=0
  Constant2 : Constant  Value=2
  Constant3 : Constant  Value=0.11
  Gain : Gain  Gain=0.447  SaturateOnIntegerOverflow=on  OutDataTypeStr=Inherit: Same as input  ParamDataTypeStr=Inherit: Same as input
  Logical : Logic
  Memory : Memory  InitialCondition=cyc_mph(1,2)*0.447/wh_radius*fd_ratio*gb_ratio(gb_num_init)
  Memory1 : Memory  InitialCondition=1
  Product : Product  Inputs=**/  InputSameDT=on  RndMeth=Zero  SaturateOnIntegerOverflow=on  OutDataTypeStr=Inherit: Same as first input
  Relational : RelationalOperator  Operator=>  RndMeth=Nearest  InputSameDT=on
  Relational1 : RelationalOperator  Operator=<=  RndMeth=Nearest  InputSameDT=on
  Sum : Sum  InputSameDT=on  SaturateOnIntegerOverflow=on  OutDataTypeStr=Inherit: Same as first input
  Sum1 : Sum  Inputs=-+  InputSameDT=on  SaturateOnIntegerOverflow=on  OutDataTypeStr=Inherit: Same as first input
  Switch : Switch  Threshold=eps  SaturateOnIntegerOverflow=on  InputSameDT=on
  Switch1 : Switch  Threshold=eps  SaturateOnIntegerOverflow=on  InputSameDT=on
  dt : Subsystem
  Out1 : Outport
  wires:
  Product/1 -> Switch/1
  Sum/1 -> Product/3
  Gain/1 -> Product/2
  [veh_spd_a_rec] -> Sum/1, Switch/2
  Constant1/1 -> Switch/3
  Memory/1 -> Switch1/1
  Constant/1 -> Sum/2
  [cyc_mph_r] -> Sum1/2
  [mpha] -> Gain/1, Sum1/1
  Constant2/1 -> Relational/2
  Sum1/1 -> Relational/1
  Relational/1 -> Memory1/1
  Switch/1 -> Memory/1
  Switch1/1 -> Out1/1
  gb_spd_in_r if no gear change/1 -> Switch1/3
  [gb_spd_in_a] -> Product/1
  Constant3/1 -> Relational1/2
  Relational1/1 -> Logical/2
  Memory1/1 -> Logical/1
  Logical/1 -> Switch1/2
  dt/1(Out1) -> Relational1/1

== system BD_PAR_SS/<vc> par/pre-TX parallel gearbox control/shifting1 ==
  gear number : Inport
  Constant : Constant  Value=gb_shift_delay-1e-6
  Relational Operator : RelationalOperator  Operator=<  RndMeth=Nearest  InputSameDT=on
  time since last shift : Subsystem
      mask Display: disp('time since\nlast shift')
  out_1 : Outport  InitialOutput=0
  wires:
  time since last shift/1(out_1) -> Relational Operator/1
  Constant/1 -> Relational Operator/2
  gear number/1 -> time since last shift/1(in_1)
  Relational Operator/1 -> out_1/1

== system BD_PAR_SS/<vc> par/pre-TX parallel gearbox control/upshift  command ==
  prev gear number : Inport
  engine load : Inport  Port=2
  engine speed : Inport  Port=3
  Mux : Mux  Inputs=2
  Relational Operator : RelationalOperator  Operator=<  RndMeth=Nearest  InputSameDT=on
  load fraction : Subsystem  mask(Gear Selector){spd=gb_upshift_spd, load=gb_upshift_load}
      mask prompts: spd "Speeds:"; load "Load Fractions:"
      mask help:
      | This block will perform a linear interplation (extrapolation outside of bounds) to determine the shift point load fraction associated with the current gear number and speed.
      |
      | The Speeds parameter should be defined as an array of vectors containing speeds for each gear number.  The Load Fractions parameter should be defined as a array of vectors containing load fractions indexed by the speeds in the Speeds parameter for each gear number.
      mask Help:
      | Reference the base workspace variables - gb_**shift_spd and gb_**shift_load  where ** is either up for upshift conditions or dn for downshift conditions.
      | 
      | Or define the arrays as follows:
      | 
      | {[spd1 spd2 spd3 spd4]; [spd1 spd2 spd3 spd4]; ...}
      | 
      | {[load1 load2 load3 load4]; [load1 load2 load3 load4]; ...}
      | 
      | where each array contains one row for each gear in the gearbox.  Speeds should be defined in rad/s and loads as a decimal fraction.
  command : Outport  InitialOutput=0
  wires:
  Relational Operator/1 -> command/1
  engine speed/1 -> Mux/2
  Mux/1 -> load fraction/1(In1)
  prev gear number/1 -> Mux/1
  engine load/1 -> Relational Operator/1
  load fraction/1(Out1) -> Relational Operator/2

== system BD_PAR_SS/<vc> par/startStop/checkAirCond ==
  air_cond_speed : Inport  OutDataTypeStr=fixdt(0,2,1,0)
  state_of_charge : Inport  Port=2
  Constant : Constant  Value=0  OutDataTypeStr=fixdt(0,1,1,0)
  Constant1 : Constant  OutDataTypeStr=fixdt(0,1,1,0)
  Logical Operator : Logic  Operator=NAND  AllPortsSameDT=off  OutDataTypeStr=fixdt(0,1,1,0)
  Switch : Switch  Threshold=3  OutDataTypeStr=fixdt(0,1,1,0)
  Switch1 : Switch  Threshold=0.7  OutDataTypeStr=fixdt(0,1,1,0)
  air_cond_check : Outport
  wires:
  Logical Operator/1 -> air_cond_check/1
  Switch/1 -> Logical Operator/1
  Switch1/1 -> Logical Operator/2
  state_of_charge/1 -> Switch1/2
  air_cond_speed/1 -> Switch/2
  Constant1/1 -> Switch1/1, Switch/1
  Constant/1 -> Switch/3, Switch1/3

== system BD_PAR_SS/<vc> par/startStop/checkBattery ==
  state_of_charge : Inport
  Constant : Constant  Value=0  OutDataTypeStr=fixdt(0,1,1,0)
  Constant1 : Constant  OutDataTypeStr=fixdt(0,1,1,0)
  Switch : Switch  Criteria=u2 > Threshold  Threshold=0.5  OutDataTypeStr=fixdt(0,1,1,0)
  To Workspace : ToWorkspace  VariableName=ss_state_of_charge  SampleTime=-1
  battery_check : Outport
  wires:
  Switch/1 -> battery_check/1
  state_of_charge/1 -> Switch/2, To Workspace/1
  Constant/1 -> Switch/3
  Constant1/1 -> Switch/1

== system BD_PAR_SS/<vc> par/startStop/checkBrake ==
  braking_status : Inport  OutDataTypeStr=fixdt(0,1,1,0)
  time : Inport  Port=2  OutDataTypeStr=fixdt(0,16,1,0)
  Switch : Switch  Threshold=1  OutDataTypeStr=fixdt(0,1,1,0)
  To Workspace : ToWorkspace  VariableName=ss_braking_status  SampleTime=-1
  checkBrakingElapsedTime : Subsystem
  brake_check : Outport
  wires:
  braking_status/1 -> checkBrakingElapsedTime/2(braking_status), To Workspace/1, Switch/3, Switch/2
  time/1 -> checkBrakingElapsedTime/1(time)
  checkBrakingElapsedTime/1(check_braking_elapsed_time) -> Switch/1
  Switch/1 -> brake_check/1

== system BD_PAR_SS/<vc> par/startStop/checkEngineTemp ==
  engine_internal_temp : Inport
  Constant : Constant  Value=0  OutDataTypeStr=fixdt(0,1,1,0)
  Constant1 : Constant  OutDataTypeStr=fixdt(0,1,1,0)
  Logical Operator : Logic  AllPortsSameDT=off  OutDataTypeStr=fixdt(0,1,1,0)
  Switch : Switch  Criteria=u2 > Threshold  Threshold=90  OutDataTypeStr=fixdt(0,1,1,0)
  Switch2 : Switch  Threshold=104  OutDataTypeStr=fixdt(0,1,1,0)
  To Workspace : ToWorkspace  VariableName=ss_engine_internal_temp  SampleTime=-1
  engine_temp_check : Outport
  wires:
  Logical Operator/1 -> engine_temp_check/1
  engine_internal_temp/1 -> To Workspace/1, Switch/2, Switch2/2
  Constant/1 -> Switch2/1, Switch/3
  Constant1/1 -> Switch2/3, Switch/1
  Switch/1 -> Logical Operator/1
  Switch2/1 -> Logical Operator/2

== system BD_PAR_SS/<vc> par/startStop/checkHardware ==
  start_stop_sensor_status : Inport  OutDataTypeStr=fixdt(0,1,1,0)
  speed_sensor_status : Inport  Port=2  OutDataTypeStr=fixdt(0,1,1,0)
  brake_sensor_status : Inport  Port=3  OutDataTypeStr=fixdt(0,1,1,0)
  engine_temp_sensor_status : Inport  Port=4  OutDataTypeStr=fixdt(0,1,1,0)
  battery_sensor_status : Inport  Port=5  OutDataTypeStr=fixdt(0,1,1,0)
  hood_sensor_status : Inport  Port=6  OutDataTypeStr=fixdt(0,1,1,0)
  trunk_sensor_status : Inport  Port=7  OutDataTypeStr=fixdt(0,1,1,0)
  door_sensor_status : Inport  Port=8  OutDataTypeStr=fixdt(0,1,1,0)
  seatbelt_sensor_status : Inport  Port=9  OutDataTypeStr=fixdt(0,1,1,0)
  air_cond_sensor_status : Inport  Port=10  OutDataTypeStr=fixdt(0,1,1,0)
  Logical Operator : Logic  Inputs=5  AllPortsSameDT=off  OutDataTypeStr=fixdt(0,1,1,0)
  Logical Operator1 : Logic  AllPortsSameDT=off  OutDataTypeStr=fixdt(0,1,1,0)
  OR : Logic  Operator=OR  Inputs=5  AllPortsSameDT=off  OutDataTypeStr=fixdt(0,1,1,0)
  hardware_status : Outport
  wires:
  speed_sensor_status/1 -> Logical Operator/2
  brake_sensor_status/1 -> Logical Operator/3
  engine_temp_sensor_status/1 -> Logical Operator/4
  battery_sensor_status/1 -> Logical Operator/5
  hood_sensor_status/1 -> OR/1
  trunk_sensor_status/1 -> OR/2
  door_sensor_status/1 -> OR/3
  seatbelt_sensor_status/1 -> OR/4
  air_cond_sensor_status/1 -> OR/5
  Logical Operator1/1 -> hardware_status/1
  Logical Operator/1 -> Logical Operator1/1
  OR/1 -> Logical Operator1/2
  start_stop_sensor_status/1 -> Logical Operator/1

== system BD_PAR_SS/<vc> par/startStop/checkSafety ==
  hood_sensor_value : Inport  OutDataTypeStr=fixdt(0,1,1,0)
  trunk_sensor_value : Inport  Port=2  OutDataTypeStr=fixdt(0,1,1,0)
  door_sensor_value : Inport  Port=3  OutDataTypeStr=fixdt(0,1,1,0)
  seatbelt_sensor_value : Inport  Port=4  OutDataTypeStr=fixdt(0,1,1,0)
  OR : Logic  Operator=OR  Inputs=4  AllPortsSameDT=off  OutDataTypeStr=fixdt(0,1,1,0)
  safety_check : Outport
  wires:
  hood_sensor_value/1 -> OR/1
  OR/1 -> safety_check/1
  trunk_sensor_value/1 -> OR/2
  door_sensor_value/1 -> OR/3
  seatbelt_sensor_value/1 -> OR/4

== system BD_PAR_SS/<vc> par/startStop/checkSpeed ==
  vehicle_speed_mph : Inport
  Constant : Constant  OutDataTypeStr=fixdt(0,1,1,0)
  Constant1 : Constant  Value=0  OutDataTypeStr=fixdt(0,1,1,0)
  Switch : Switch  Threshold=5  OutDataTypeStr=fixdt(0,1,1,0)
  To Workspace2 : ToWorkspace  VariableName=ss_vehicle_speed_mph  SampleTime=-1
  mph --> km/h : Gain  Gain=1.6095
  speed_check : Outport
  wires:
  Switch/1 -> speed_check/1
  mph --> km/h/1 -> Switch/2
  vehicle_speed_mph/1 -> To Workspace2/1, mph --> km/h/1
  Constant1/1 -> Switch/1
  Constant/1 -> Switch/3

== system BD_PAR_SS/<vc> par/startStop/checkSystemLatency ==
  start_stop_status : Inport
  engine_status : Inport  Port=2  OutDataTypeStr=fixdt(0,1,1,0)
  time : Inport  Port=3
  Constant2 : Constant  Value=0  OutDataTypeStr=fixdt(0,1,1,0)
  Logical Operator : Logic  Operator=NOR  AllPortsSameDT=off  OutDataTypeStr=fixdt(0,1,1,0)
  Switch : Switch  Threshold=1  OutDataTypeStr=fixdt(0,1,1,0)
  checkRestartEngineElapsedTime : Subsystem
  latency_check : Outport
  wires:
  Constant2/1 -> Switch/3
  Logical Operator/1 -> Switch/2, checkRestartEngineElapsedTime/2(braking_status)
  Switch/1 -> latency_check/1
  checkRestartEngineElapsedTime/1(check_restart_engine_elapsed_time) -> Switch/1
  time/1 -> checkRestartEngineElapsedTime/1(time)
  engine_status/1 -> Logical Operator/2
  start_stop_status/1 -> Logical Operator/1

== system BD_PAR_SS/drive cycle <cyc>/distance travelled (m)/Block NOTES ==
  note: This block calculates the distance travelled by the
      |  vehicle based on the achieved speed.

== system BD_PAR_SS/drive cycle <cyc>/super-smooth, no-lag trace/Subsystem ==
  in_1 : Inport
  Constant1 : Constant  Value=n
  Integrator : Integrator
  Product : Product  Inputs=*/  InputSameDT=on  RndMeth=Zero  SaturateOnIntegerOverflow=on  OutDataTypeStr=Inherit: Same as first input
  Sum : Sum  Inputs=+-  InputSameDT=on  SaturateOnIntegerOverflow=on  OutDataTypeStr=Inherit: Same as first input
  Transport Delay : TransportDelay  DelayTime=n
  out_1 : Outport  InitialOutput=0
  wires:
  Integrator/1 -> Sum/1, Transport Delay/1
  Transport Delay/1 -> Sum/2
  Sum/1 -> Product/1
  in_1/1 -> Integrator/1
  Product/1 -> out_1/1
  Constant1/1 -> Product/2

== system BD_PAR_SS/drive cycle <cyc>/super-smooth, no-lag trace/repeated cycle ==
  Clock : Clock
  Fcn1 : Fcn  Expr=rem(u+avgtime*0.75,period)
  Look-Up Table : Lookup  InputValues=t  Table=y  SaturateOnIntegerOverflow=on
  out_1 : Outport  InitialOutput=0
  wires:
  Fcn1/1 -> Look-Up Table/1
  Clock/1 -> Fcn1/1
  Look-Up Table/1 -> out_1/1

== system BD_PAR_SS/electric acc loads <acc>/Electrical Accessory Loads v2 <acc>/Accessory SDO ==
  data bus : Inport
  Demux : Demux  Outputs=3
      settings: DisplayOption=none
  To Workspace : ToWorkspace  VariableName=acc_elec_pwr_r  SampleTime=-1
  To Workspace3 : ToWorkspace  VariableName=acc_elec_pwr_a  SampleTime=-1
  To Workspace4 : ToWorkspace  VariableName=acc_elec_pwr_est  SampleTime=-1
  electrical power logging : Subsystem  mask{eff=acc_mech_eff}
      mask prompts: eff "efficiency of accessory systems (decimal)"
  wires:
  Demux/3 -> To Workspace4/1
  Demux/2 -> electrical power logging/1(In1), To Workspace3/1
  Demux/1 -> To Workspace/1
  data bus/1 -> Demux/1

== system BD_PAR_SS/electric acc loads <acc>/Electrical Accessory Loads v2 <acc>/Block NOTES ==
  note: This is the electrical auxiliary loads model.
  note: In terms of an interface, the model assumes electrical power generated from
      | a powersource (or powersources)
      |
      | This model takes in requested driveline electrical power output requests and
      | augments power to account for electrically driven accessories.
      |
      | The power passed along down to the driveline is only power to move the
      | vehicle.

== system BD_PAR_SS/electric acc loads <acc>/Electrical Accessory Loads v2 <acc>/backward model ==
  note: Power Electrical
      | Accessory
      | (W)
  note: P, W, for driveline
  note: Pwr, W, powersource out
  pwr_in : Inport
  on/off : Inport  Port=2
  Constant : Constant  Value=load_on
  Product : Product  Inputs=***  InputSameDT=on  RndMeth=Zero  SaturateOnIntegerOverflow=on  OutDataTypeStr=Inherit: Same as first input
  Sum : Sum  Inputs=|++  InputSameDT=on  SaturateOnIntegerOverflow=on  OutDataTypeStr=Inherit: Same as first input
  electrical accessories (W) : Subsystem  BlockChoice=Electrical Accessories: Time Variable
      settings: AttributesFormatString=%<BlockChoice>  TemplateBlock=lib_accessory/electrical accessories (W)  MemberBlocks=Electrical Accessories: Constant,Electrical Accessories: Time Variable
      mask Display: image(imread('bdi_acc_elec_cs.bmp'))
  elec_out : Outport
  elec_acc_out : Outport  Port=2
  wires:
  Product/1 -> Sum/2, elec_acc_out/1
  Constant/1 -> Product/3
  on/off/1 -> Product/2
  electrical accessories (W)/1(P_elec_acc) -> Product/1
  pwr_in/1 -> Sum/1
  Sum/1 -> elec_out/1

== system BD_PAR_SS/electric acc loads <acc>/Electrical Accessory Loads v2 <acc>/forward model ==
  note: ASSUMPTIONS
  note: This calculation assumes that the power provider is never so power limited as to
      | not be able to provide at least the value of acc_pwr_in.
  note: electric
      | accessory
      | power (W)
  note: Power Available
  note: Power to driveline
  pwr_in : Inport
  acc_pwr_in : Inport  Port=2
  Sum : Sum  Inputs=|+-  InputSameDT=on  SaturateOnIntegerOverflow=on  OutDataTypeStr=Inherit: Same as first input
  pwr_out : Outport
  acc_pwr_out : Outport  Port=2
  wires:
  acc_pwr_in/1 -> acc_pwr_out/1, Sum/2
  pwr_in/1 -> Sum/1
  Sum/1 -> pwr_out/1
